simulink model "logistic_map"  (R2023b)
settings: Solver=FixedStepAuto  StartTime=0.0  StopTime=100  FixedStep=1  RelTol=1e-3
settings Model: Creator=vaclav  LastModifiedBy=vaclav
settings OptimizationCC: ReuseModelBlockBuffer=off

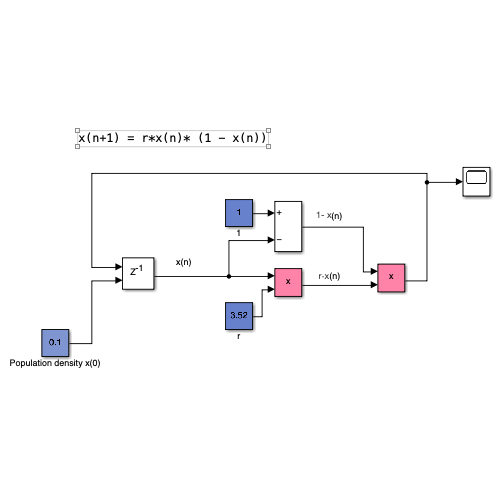
[thumbnail: Simulink's stored preview of the top-level diagram]
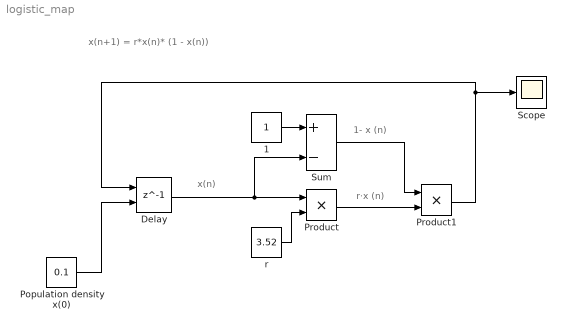
== system logistic_map ==
  note: x(n)
  note: x(n+1) = r*x(n)* (1 - x(n))
  note: r⋅x (n)
  note: 1- x (n)
  1 : Constant
  Delay : Delay  DelayLength=1  InitialConditionSource=Input port
      settings: InputPortMap=u0,p4
  Population density x(0) : Constant  Value=0.1
  Product : Product
  Product1 : Product
  Scope : Scope
  Sum : Sum  Inputs=+-
  r : Constant  Value=3.52
  wires:
  Population density x(0)/1 -> Delay/2
  Delay/1 -> Sum/2, Product/1
  r/1 -> Product/2
  Product/1 -> Product1/2
  1/1 -> Sum/1
  Product1/1 -> Scope/1, Delay/1
  Sum/1 -> Product1/1
